simulink model "simple_block_diagram"  (R2015a)
settings: Solver=ode45  StartTime=0.0  StopTime=10.0  RelTol=1e-3
settings Model: Creator=ayush  LastModifiedBy=ayush

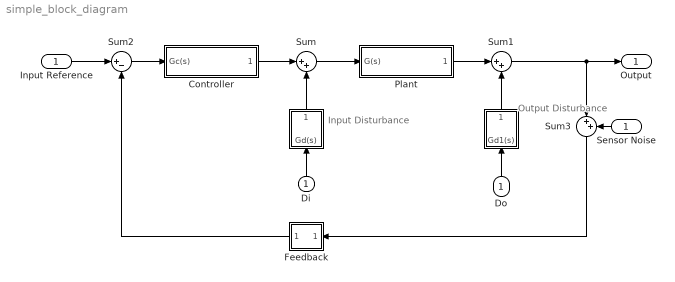
== system simple_block_diagram ==
  note: Input
      | Disturbance
  note: Output
      | Disturbance
  Input Reference : Inport
  " " : Subsystem
  "  " : Subsystem
  " Di" : InportShadow
  Controller : Subsystem
  Do : InportShadow
  Feedback : Subsystem
  Plant : Subsystem
  Sensor Noise : InportShadow
  Sum : Sum  Inputs=|++
  Sum1 : Sum  Inputs=|++
  Sum2 : Sum  Inputs=|+-
  Sum3 : Sum  Inputs=|++
  Output : Outport
  wires:
  Controller/1(" ") -> Sum/1
  Sum/1 -> Plant/1("\t\t\t\t\t\t\t\t\t\t\t\t\t\tG(s)")
  Plant/1(" ") -> Sum1/1
  " "/1(" ") -> Sum/2
  "  "/1(" ") -> Sum1/2
  Sum2/1 -> Controller/1("\t\t\t\t\t\t\t\t\t\t\t\t\t\tGc(s)")
  Sum1/1 -> Output/1, Sum3/1
  Input Reference/1 -> Sum2/1
  Sum3/1 -> Feedback/1("                \t\t\t\t\t\t\t\t\t\t\t\t \t\t\t\t\t\t\t\t\t\t\t H(s)")
  Sensor Noise/1 -> Sum3/2
  Feedback/1(" ") -> Sum2/2
  Do/1 -> "  "/1(Gd1(s))
  " Di"/1 -> " "/1(Gd(s))

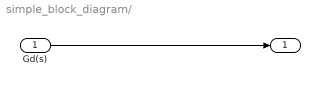
== system simple_block_diagram/  ==
  Gd(s) : Inport
  " " : Outport
  wires:
  Gd(s)/1 -> " "/1

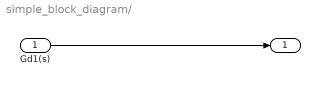
== system simple_block_diagram/   ==
  Gd1(s) : Inport
  " " : Outport
  wires:
  Gd1(s)/1 -> " "/1

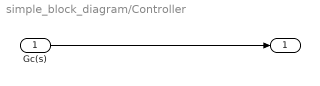
== system simple_block_diagram/Controller ==
  "\t\t\t\t\t\t\t\t\t\t\t\t\t\tGc(s)" : Inport
  " " : Outport
  wires:
  "\t\t\t\t\t\t\t\t\t\t\t\t\t\tGc(s)"/1 -> " "/1

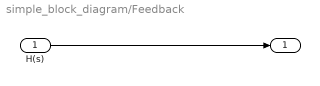
== system simple_block_diagram/Feedback ==
  "                \t\t\t\t\t\t\t\t\t\t\t\t \t\t\t\t\t\t\t\t\t\t\t H(s)" : Inport
  " " : Outport
  wires:
  "                \t\t\t\t\t\t\t\t\t\t\t\t \t\t\t\t\t\t\t\t\t\t\t H(s)"/1 -> " "/1

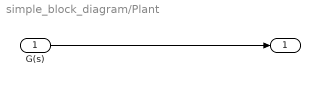
== system simple_block_diagram/Plant ==
  "\t\t\t\t\t\t\t\t\t\t\t\t\t\tG(s)" : Inport
  " " : Outport
  wires:
  "\t\t\t\t\t\t\t\t\t\t\t\t\t\tG(s)"/1 -> " "/1
